simulink model "L_27_04_21_esempio_ok"  (R2021a)
settings: Solver=VariableStepAuto  StartTime=0.0  StopTime=20.0  RelTol=1e-6
values from neighbouring files (symbols this model uses):
  Kc = Kr/(Kf*0.2)    [L_11_05_21_reti_anticipatrici.m]    (also in L_11_05_21_reti_anticipatrici_2.m; L_12_05_21_Esercizio_progetto_di_un_controllore.m = 1/(0.04*Kf1*Kf2); L_12_05_21_effetti_sul_comando.m = 4; L_12_05_21_reti_integro-derivative.m = 4)
  Kr = 1    [L_11_05_21_reti_anticipatrici.m]    (also in L_11_05_21_reti_anticipatrici_2.m; L_12_05_21_Esercizio_progetto_di_un_controllore.m; L_12_05_21_effetti_sul_comando.m; L_12_05_21_reti_integro-derivative.m)
libraries: cstblocks x1, simulink x1
settings Model: Creator=fornasierarmando  LastModifiedBy=fornasierarmando

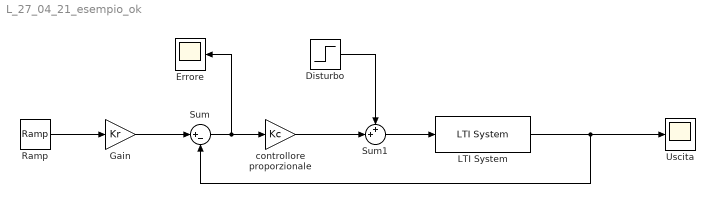
== system L_27_04_21_esempio_ok ==
  Disturbo : Step  Time=0  After=0  SampleTime=0
  Errore : Scope
  Gain : Gain  Gain=Kr
  "LTI System " : cstblocks/LTI System  sys=F  IC=[]
  Ramp : simulink/Sources/Ramp  slope=1  start=0  InitialOutput=0
  Sum : Sum  Inputs=|+-
  Sum1 : Sum  Inputs=++|
  Uscita : Scope
  controllore proporzionale : Gain  Gain=Kc
  wires:
  Disturbo/1 -> Sum1/1
  Ramp/1 -> Gain/1
  controllore proporzionale/1 -> Sum1/2
  Sum1/1 -> "LTI System "/1
  "LTI System "/1 -> Sum/2, Uscita/1
  Sum/1 -> controllore proporzionale/1, Errore/1
  Gain/1 -> Sum/1
